simulink model "rgps_model"  (R2020a)
settings: Solver=FixedStepAuto  StartTime=0.0  StopTime=5600  FixedStep=112  RelTol=1e-3
settings Model: Creator=lu  LastModifiedBy=utente
settings DataIOCC: ReturnWorkspaceOutputs=off
settings DebuggingCC: ArithmeticOperatorsInVariantConditions=warning
settings SFSimCC: CustomCodeUndefinedFunction=UseInterfaceOnly

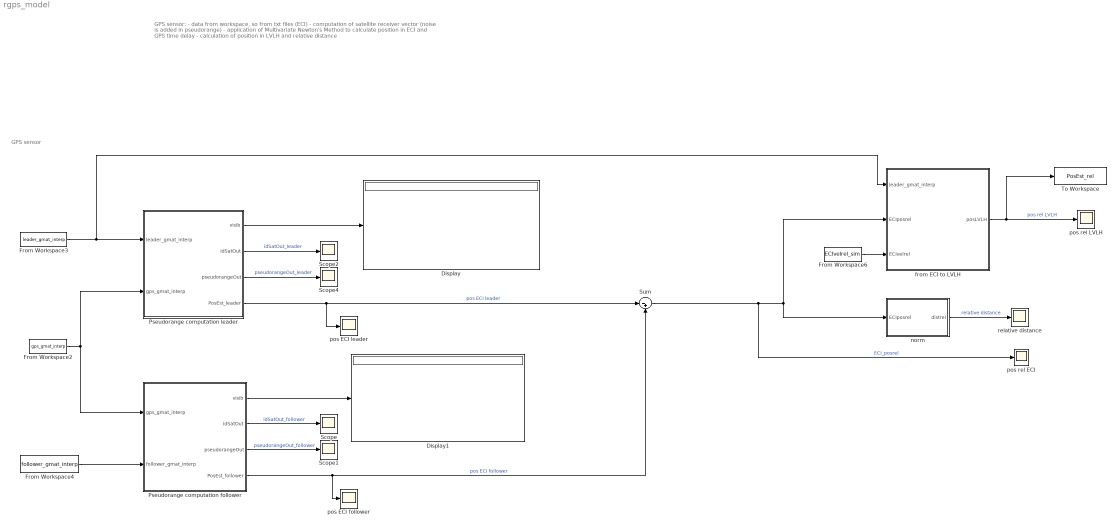
== system rgps_model ==
  note: GPS sensor
  note: GPS sensor:
      | - data from workspace, so from txt files (ECI)
      | - computation of satellite receiver vector (noise is added in pseudorange)
      | - application of Multivariate Newton's Method to calculate position in ECI and GPS time delay
      | - calculation of position in LVLH and relative distance
  Display : Display
  Display1 : Display
  From Workspace2 : FromWorkspace  VariableName=gps_gmat_interp
  From Workspace3 : FromWorkspace  VariableName=leader_gmat_interp
  From Workspace4 : FromWorkspace  VariableName=follower_gmat_interp
  From Workspace6 : FromWorkspace  VariableName=ECIvelrel_sim
  Pseudorange computation follower : MATLAB Function  TreatAsAtomicUnit=on
  Pseudorange computation leader : MATLAB Function  TreatAsAtomicUnit=on
  Scope{,1..2,4} (4 alike) : Scope
  Sum : Sum  Inputs=|-+
  To Workspace : ToWorkspace  VariableName=PosEst_rel  SaveFormat=Timeseries  SampleTime=-1
  from ECI to LVLH : MATLAB Function  TreatAsAtomicUnit=on
  "norm " : MATLAB Function  TreatAsAtomicUnit=on
  pos ECI follower : Scope
  pos ECI leader : Scope
  pos rel ECI : Scope
  pos rel LVLH : Scope
  relative distance : Scope
  wires:
  From Workspace4/1 -> Pseudorange computation follower/2(follower_gmat_interp)
  Pseudorange computation leader/3(pseudorangeOut) -> Scope4/1  "pseudorangeOut_leader"
  From Workspace2/1 -> Pseudorange computation follower/1(gps_gmat_interp), Pseudorange computation leader/2(gps_gmat_interp)
  Pseudorange computation follower/1(visib) -> Display1/1
  Pseudorange computation leader/2(idSatOut) -> Scope2/1  "idSatOut_leader"
  Pseudorange computation follower/2(idSatOut) -> Scope/1  "idSatOut_follower"
  From Workspace6/1 -> from ECI to LVLH/3(ECIvelrel)
  From Workspace3/1 -> from ECI to LVLH/1(leader_gmat_interp), Pseudorange computation leader/1(leader_gmat_interp)
  Pseudorange computation leader/1(visib) -> Display/1
  "norm "/1(distrel) -> relative distance/1  "relative distance"
  Pseudorange computation follower/4(PosEst_follower) -> Sum/2, pos ECI follower/1  "pos ECI follower"
  from ECI to LVLH/1(posLVLH) -> To Workspace/1, pos rel LVLH/1  "pos rel LVLH"
  Sum/1 -> "norm "/1(ECIposrel), from ECI to LVLH/2(ECIposrel), pos rel ECI/1  "ECI_posrel"
  Pseudorange computation follower/3(pseudorangeOut) -> Scope1/1  "pseudorangeOut_follower"
  Pseudorange computation leader/4(PosEst_leader) -> Sum/1, pos ECI leader/1  "pos ECI leader"

== matlab function rgps_model/Pseudorange computation follower ==
  data: gps_gmat_interp input; visib output; follower_gmat_interp input; idSatOut output; pseudorangeOut output; PosEst_follower output
function [visib, idSatOut, pseudorangeOut, PosEst_follower]   = fcn(gps_gmat_interp, follower_gmat_interp)

totsat=24;
c=299792.458; %speed of light [km/s]

% FOLLOWER

numsat = 0; % number of visible gps satellite
visib = zeros(1,totsat); % visibility vector
dist = zeros(1,totsat); % distance between gps satellite and follower
elev = zeros(1,totsat); % gps satellite elevation
pseudorange = zeros(1,totsat); % pseudorange from gps satellite
idSat = zeros(1,totsat); % identification of gps satellite
tt=zeros(1,totsat); % trasmission time

for satellite = 1:totsat
    % Extract position of i-th gps satellite
    posSat = gps_gmat_interp(3*(satellite-1)+1:3*(satellite-1)+3,:);    
    
    % computation of gps satellite receiver vector
    sl = posSat-follower_gmat_interp;
    dist(satellite) = norm(sl);
    hSat = follower_gmat_interp'/norm(follower_gmat_interp)*sl;
    elev(satellite) = asin(hSat/norm(sl));
    
    % visibility of gps satellite
    if hSat > 0 && elev(satellite) >= 5*pi/180
        visib(satellite) = 1; % is visible
        numsat=numsat+1; % update n° of gps visible sat
        pseudorange(numsat) = dist(satellite)+randi([-0.05,0.05]); % update pseudoranges     
        idSat(numsat) = satellite;
        tt(numsat)=pseudorange(numsat)/c;
    else
        visib(satellite) = 0;
    end
end
idSatOut = idSat(1:4);
pseudorangeOut = pseudorange(1:4);
ttOut=tt(1:4);

%% solution (Multivariate Newton's Method)
% ref: http://mason.gmu.edu/~nulloaso/Project2.html

% position of gps visible satellites (4 sats needed)
PsatVis = zeros(3,4);
for nsat = 1:4
    PsatVis(:,nsat)=gps_gmat_interp(3*(idSatOut(nsat)-1)+1:3*(idSatOut(nsat)-1)+3);
end

% simultaneous gps satellite positions [km]
A1= PsatVis(1,1); B1= PsatVis(2,1); C1= PsatVis(3,1);
A2 = PsatVis(1,2); B2= PsatVis(2,2); C2=PsatVis(3,2);
A3 = PsatVis(1,3); B3 = PsatVis(2,3); C3= PsatVis(3,3);
A4= PsatVis(1,4); B4=PsatVis(2,4); C4=PsatVis(3,4);

% trasmission time intervals [s]
t1= ttOut(1);
t2= ttOut(2);
t3= ttOut(3);
t4= ttOut(4);

% initial vector
u= [0;0;6370+400;0]; % [x_eci y_eci z_eci time_delay] guess values, they may depend on true trajectories

x=zeros(1,10);
y=zeros(1,10);
z=zeros(1,10);
d=zeros(1,10);

% iteration
for i=1: 10
   
    x(i)= u(1);
    y(i)= u(2) ;
    z(i)= u(3);
    d(i)= u(4);
    
    % functions of (x,y,z,d), from (4.73)
    f1= ( x(i)-A1).^2 + (y(i)-B1).^2 + (z(i)-C1).^2 - (c*(t1 - d(i))).^2;
    f2= ( x(i)-A2).^2 + (y(i)-B2).^2 + (z(i)-C2).^2 - (c*(t2 - d(i))).^2;
    f3= ( x(i)-A3).^2 + (y(i)-B3).^2 + (z(i)-C3).^2 - (c*(t3 - d(i))).^2;
    f4= ( x(i)-A4).^2 + (y(i)-B4).^2 + (z(i)-C4).^2 - (c*(t4 - d(i))).^2; 
    F = [f1;f2;f3;f4];
   
   % Jacobian Matrix
   df1x= (2*(x(i)-A1));
   df1y= (2*(y(i)-B1));
   df1z= (2*(z(i)-C1));
   df1t= (2*c^2*(t1-d(i)));
 
   df2x=2*(x(i)-A2);
   df2y=2*(y(i)-B2);
   df2z=2*(z(i)-C2);
   df2t=2*c^2*(t2-d(i));

   df3x=2*(x(i)-A3);
   df3y=2*(y(i)-B3);
   df3z=2*(z(i)-C3);
   df3t=2*c^2*(t3-d(i));

   df4x=2*(x(i)-A4);
   df4y=2*(y(i)-B4);
   df4z=2*(z(i)-C4);
   df4t=2*c^2*(t4-d(i));

   DF = [df1x, df1y, df1z, df1t; df2x, df2y df2z df2t;df3x df3y df3z df3t;df4x df4y df4z df4t];
   
   % new u(x,y,z,d) vector
    V = DF\(-F);
    u = u+V;

end

PosEst_follower=u;

== matlab function rgps_model/Pseudorange computation leader ==
  data: leader_gmat_interp input; gps_gmat_interp input; visib output; idSatOut output; pseudorangeOut output; PosEst_leader output
function [visib, idSatOut, pseudorangeOut, PosEst_leader]   = fcn(leader_gmat_interp, gps_gmat_interp)

totsat=24;
c=3*10^8; % [m/s]

% LEADER

numsat = 0; % number of visible gps satellite
visib = zeros(1,totsat); % visibility vector
dist = zeros(1,totsat); % distance between gps satellite and follower
elev = zeros(1,totsat); % gps satellite elevation
pseudorange = zeros(1,totsat); % pseudorange from gps satellite
idSat = zeros(1,totsat); % identification of gps satellite
tt=zeros(1,totsat); % trasmission time (affected by time delay)

for satellite = 1:1:totsat
    % Extract position of i-th gps satellite
    posSat = gps_gmat_interp(3*(satellite-1)+1:3*(satellite-1)+3); % [3x1]
    
    % computation of gps satellite receiver vector
    sl = posSat-leader_gmat_interp; % [3x1]
    dist(satellite) = norm(sl);
    hSat = leader_gmat_interp'/norm(leader_gmat_interp)*sl;
    elev(satellite) = asin(hSat/norm(sl));
    
    % visibility of gps satellite
    if hSat > 0 && elev(satellite) >= 5*pi/180
        visib(satellite) = 1; % is visible
        numsat=numsat+1; % update n° of visible gps sats
        pseudorange(numsat) = dist(satellite)+randi([-0.05,0.05]); % update pseudoranges     
        idSat(numsat) = satellite;
        tt(numsat)=pseudorange(numsat)/c;
    end
end

idSatOut = idSat(1:4);
pseudorangeOut = pseudorange(1:4);
ttOut=tt(1:4);
%% Solution (Multivariate Newton's Method)
%ref: http://mason.gmu.edu/~nulloaso/Project2.html

% position of visible gps satellites (4 sats needed)
PsatVis = zeros(3,4);
for nsat = 1:4
    PsatVis(:,nsat)=gps_gmat_interp(3*(idSatOut(nsat)-1)+1:3*(idSatOut(nsat)-1)+3);
end

% simultaneous gps satellite positions [km]
A1= PsatVis(1,1); B1= PsatVis(2,1); C1= PsatVis(3,1);
A2 = PsatVis(1,2); B2= PsatVis(2,2); C2=PsatVis(3,2);
A3 = PsatVis(1,3); B3 = PsatVis(2,3); C3= PsatVis(3,3);
A4= PsatVis(1,4); B4=PsatVis(2,4); C4=PsatVis(3,4);

% trasmission time intervals [s]
t1= ttOut(1);
t2= ttOut(2);
t3= ttOut(3);
t4= ttOut(4);

% initial vector
u= [0;0;6370+400;0]; % [x_eci y_eci z_eci time_delay] guess values, they may depend on true trajectories

x=zeros(1,10);
y=zeros(1,10);
z=zeros(1,10);
d=zeros(1,10);

% iteration
for i=1: 10
   
    x(i)= u(1);
    y(i)= u(2);
    z(i)= u(3);
    d(i)= u(4);
    
    % functions of (x,y,z,d), from (4.73)
    f1= ( x(i)-A1).^2 + (y(i)-B1).^2 + (z(i)-C1).^2 - (c*(t1 - d(i))).^2;
    f2= ( x(i)-A2).^2 + (y(i)-B2).^2 + (z(i)-C2).^2 - (c*(t2 - d(i))).^2;
    f3= ( x(i)-A3).^2 + (y(i)-B3).^2 + (z(i)-C3).^2 - (c*(t3 - d(i))).^2;
    f4= ( x(i)-A4).^2 + (y(i)-B4).^2 + (z(i)-C4).^2 - (c*(t4 - d(i))).^2; 
    F = [f1;f2;f3;f4];
   
   % Jacobian Matrix
   df1x= (2*(x(i)-A1));
   df1y= (2*(y(i)-B1));
   df1z= (2*(z(i)-C1));
   df1t= (2*c^2*(t1-d(i)));
 
   df2x=2*(x(i)-A2);
   df2y=2*(y(i)-B2);
   df2z=2*(z(i)-C2);
   df2t=2*c^2*(t2-d(i));

   df3x=2*(x(i)-A3);
   df3y=2*(y(i)-B3);
   df3z=2*(z(i)-C3);
   df3t=2*c^2*(t3-d(i));

   df4x=2*(x(i)-A4);
   df4y=2*(y(i)-B4);
   df4z=2*(z(i)-C4);
   df4t=2*c^2*(t4-d(i));

   DF = [df1x, df1y, df1z, df1t; df2x, df2y df2z df2t;df3x df3y df3z df3t;df4x df4y df4z df4t];
   
   % new u(x,y,z,d) vector
    V = DF\(-F);
    u = u+V;

end

PosEst_leader=u;

== matlab function rgps_model/from ECI to LVLH ==
  data: leader_gmat_interp input; ECIposrel input; posLVLH output; ECIvelrel input
function posLVLH = fcn(leader_gmat_interp,ECIposrel, ECIvelrel)
% transformation of reference system from ECI to LVLH


er=ECIposrel(2:end)/norm(ECIposrel(2:end)); % unit vector in r-bar
en=cross(ECIposrel(2:end), ECIvelrel)/norm(cross(ECIposrel(2:end), ECIvelrel)); % unit vector in h-bar
et=cross(er,en); % unit vector orthogonal to the others (v-bar)

posLVLH=zeros(3,1);

posLVLH(1)=ECIposrel(2)*er(1)+ECIposrel(3)*er(2)+ECIposrel(4)*er(3);
posLVLH(2)=ECIposrel(2)*en(1)+ECIposrel(3)*en(2)+ECIposrel(4)*en(3);
posLVLH(3)=ECIposrel(2)*et(1)+ECIposrel(3)*et(2)+ECIposrel(4)*et(3);


posLVLH=posLVLH+leader_gmat_interp; % traslation

== matlab function rgps_model/norm  ==
  data: ECIposrel input; distrel output
function distrel  = fcn(ECIposrel)

distrel=norm(ECIposrel);
